simulink model "untimed_ctrl_test"  (R2021b)
settings: Solver=VariableStepAuto  StartTime=0.0  StopTime=ticks-1  RelTol=1e-3
libraries: dspsrcs4 x4
settings Model: Creator=torha  LastModifiedBy=torha
settings SolverCC: AlgebraicLoopSolver=TrustRegion
settings DebuggingCC: SFMachineParentedDataDiag=warning

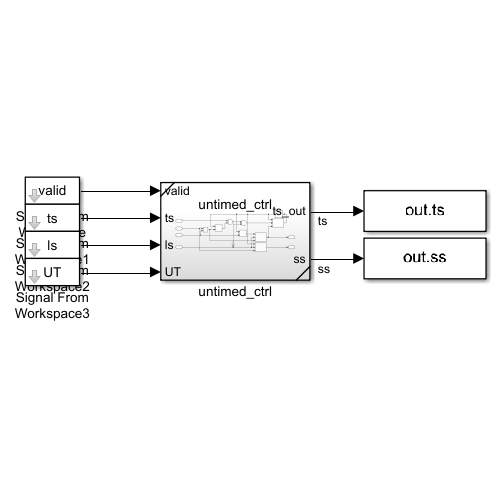
[thumbnail: Simulink's stored preview of the top-level diagram]
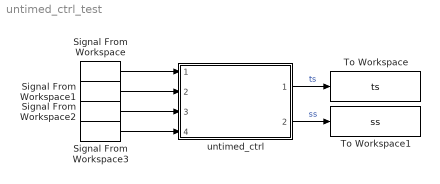
== system untimed_ctrl_test ==
  Signal From Workspace : dspsrcs4/Signal From Workspace  X=valid  Ts=1  nsamps=1  OutputAfterFinalValue=Setting to zero  ignoreOrWarnInputAndFrameLengths=off  OutputFrames=off
  Signal From Workspace1 : dspsrcs4/Signal From Workspace  X=ts  Ts=1  nsamps=1  OutputAfterFinalValue=Setting to zero  ignoreOrWarnInputAndFrameLengths=off  OutputFrames=off
  Signal From Workspace2 : dspsrcs4/Signal From Workspace  X=ls  Ts=1  nsamps=1  OutputAfterFinalValue=Setting to zero  ignoreOrWarnInputAndFrameLengths=off  OutputFrames=off
  Signal From Workspace3 : dspsrcs4/Signal From Workspace  X=UT  Ts=1  nsamps=1  OutputAfterFinalValue=Setting to zero  ignoreOrWarnInputAndFrameLengths=off  OutputFrames=off
  To Workspace : ToWorkspace  VariableName=ts  SampleTime=-1
      settings: Save2DSignal=2-D array (concatenate along first dimension)
  To Workspace1 : ToWorkspace  VariableName=ss  SampleTime=-1
      settings: Save2DSignal=2-D array (concatenate along first dimension)
  untimed_ctrl : Subsystem  ReferencedSubsystem=untimed_ctrl
  wires:
  Signal From Workspace/1 -> untimed_ctrl/1
  Signal From Workspace1/1 -> untimed_ctrl/2
  Signal From Workspace2/1 -> untimed_ctrl/3
  Signal From Workspace3/1 -> untimed_ctrl/4
  untimed_ctrl/1 -> To Workspace/1  "ts"
  untimed_ctrl/2 -> To Workspace1/1  "ss"
